simulink model "N3Sim"  (R2023b)
settings: Solver=FixedStepAuto  StartTime=0.0  StopTime=1.04  RelTol=1e-3
values from neighbouring files (symbols this model uses):
  kd = -0.0005    [N3Parameters.m]
  td = 0.01    [N3Parameters.m]
  tl1 = 0.0000199    (= 1.99e-05)    [N3Parameters.m]
  tl2 = 0.0000121    (= 1.21e-05)    [N3Parameters.m]
settings Model: Creator=olavhegg  LastModifiedBy=olavhegg

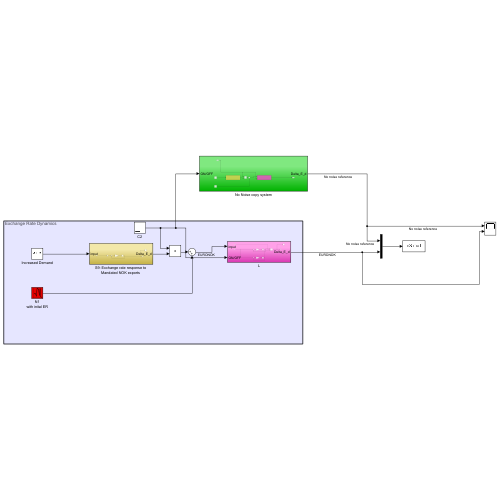
[thumbnail: Simulink's stored preview of the top-level diagram]
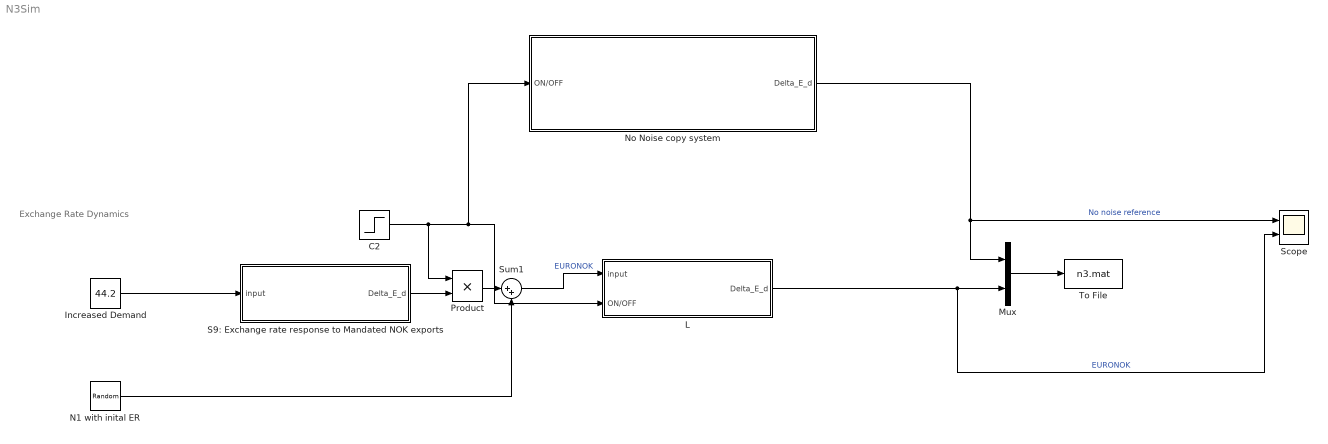
== system N3Sim ==
  note: Exchange Rate Dynamics
  C2 : Step  Time=0.1  SampleTime=0
  Increased Demand : Constant  Value=44.2
  L : Subsystem
  Mux : Mux  Inputs=2
  N1 with inital ER : RandomNumber  Mean=12  Variance=0.00001259  Seed=23341  SampleTime=0.00142857
  No Noise copy system : Subsystem
  Product : Product
  "S9: Exchange rate response to Mandated NOK exports " : Subsystem
  Scope : Scope  NumInputPorts=2
  Sum1 : Sum  Inputs=|++
  To File : ToFile  Filename=n3.mat  MatrixName=n3  SampleTime=0.0001
  wires:
  Product/1 -> Sum1/1
  N1 with inital ER/1 -> Sum1/2
  Sum1/1 -> L/1(input)  "EURONOK"
  No Noise copy system/1(Delta_E_d) -> Mux/1, Scope/1  "No noise reference"
  Mux/1 -> To File/1
  "S9: Exchange rate response to Mandated NOK exports "/1(Delta_E_d) -> Product/2
  C2/1 -> No Noise copy system/1(ON/OFF), L/2(ON/OFF), Product/1
  Increased Demand/1 -> "S9: Exchange rate response to Mandated NOK exports "/1(input)
  L/1(Delta_E_d) -> Scope/2, Mux/2  "EURONOK"

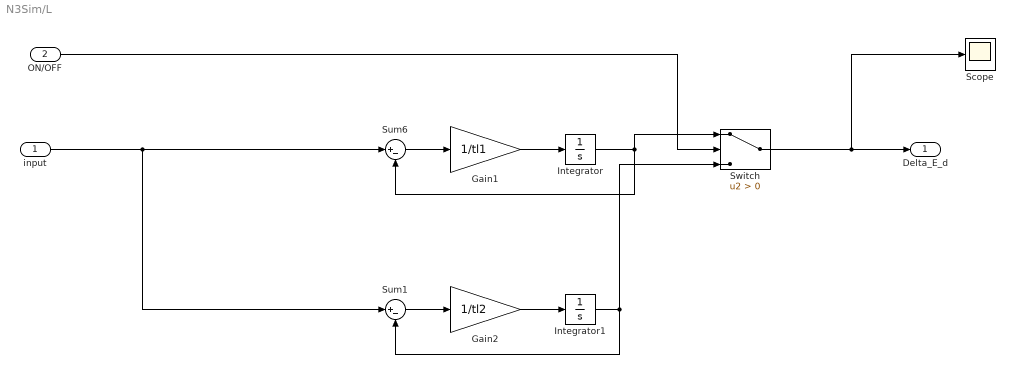
== system N3Sim/L ==
  input : Inport
  ON/OFF : Inport  Port=2
  Gain1 : Gain  Gain=1/tl1
  Gain2 : Gain  Gain=1/tl2
  Integrator : Integrator  InitialCondition=12
  Integrator1 : Integrator  InitialCondition=12
  Scope : Scope
  Sum1 : Sum  Inputs=|+-
  Sum6 : Sum  Inputs=|+-
  Switch : Switch  Criteria=u2 > Threshold  SaturateOnIntegerOverflow=off  InputSameDT=off
  Delta_E_d : Outport
  wires:
  Gain1/1 -> Integrator/1
  Sum6/1 -> Gain1/1
  Integrator/1 -> Switch/1, Sum6/2
  Integrator1/1 -> Switch/3, Sum1/2
  input/1 -> Sum1/1, Sum6/1
  Sum1/1 -> Gain2/1
  Gain2/1 -> Integrator1/1
  Switch/1 -> Scope/1, Delta_E_d/1
  ON/OFF/1 -> Switch/2

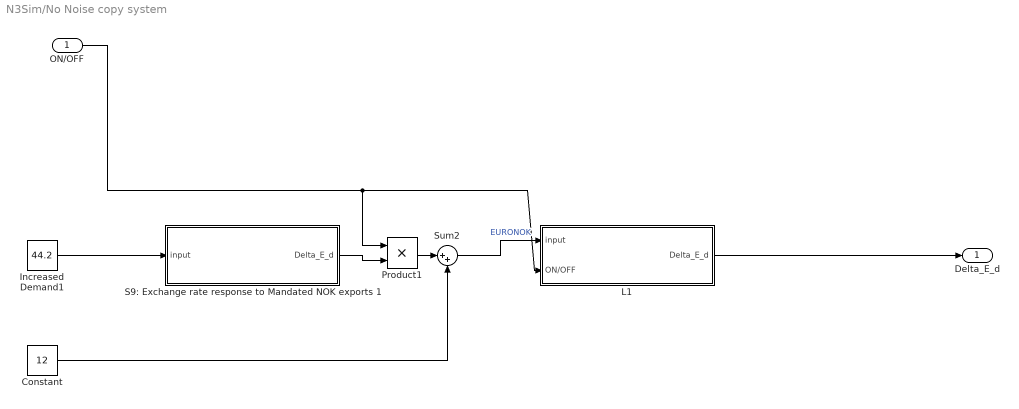
== system N3Sim/No Noise copy system ==
  ON/OFF : Inport
  Constant : Constant  Value=12
  Increased Demand1 : Constant  Value=44.2
  L1 : Subsystem
  Product1 : Product
  S9: Exchange rate response to Mandated NOK exports 1 : Subsystem
  Sum2 : Sum  Inputs=|++
  Delta_E_d : Outport
  wires:
  Increased Demand1/1 -> S9: Exchange rate response to Mandated NOK exports 1/1(input)
  ON/OFF/1 -> L1/2(ON/OFF), Product1/1
  Product1/1 -> Sum2/1
  L1/1(Delta_E_d) -> Delta_E_d/1
  Sum2/1 -> L1/1(input)  "EURONOK"
  Constant/1 -> Sum2/2
  S9: Exchange rate response to Mandated NOK exports 1/1(Delta_E_d) -> Product1/2

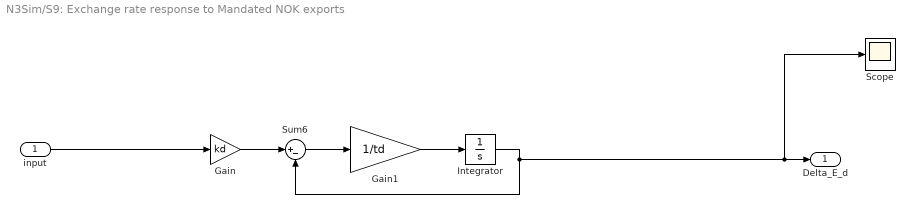
== system N3Sim/S9: Exchange rate response to Mandated NOK exports  ==
  input : Inport
  Gain : Gain  Gain=kd
  Gain1 : Gain  Gain=1/td
  Integrator : Integrator
  Scope : Scope
  Sum6 : Sum  Inputs=|+-
  Delta_E_d : Outport
  wires:
  Gain/1 -> Sum6/1
  Gain1/1 -> Integrator/1
  Sum6/1 -> Gain1/1
  input/1 -> Gain/1
  Integrator/1 -> Scope/1, Delta_E_d/1, Sum6/2

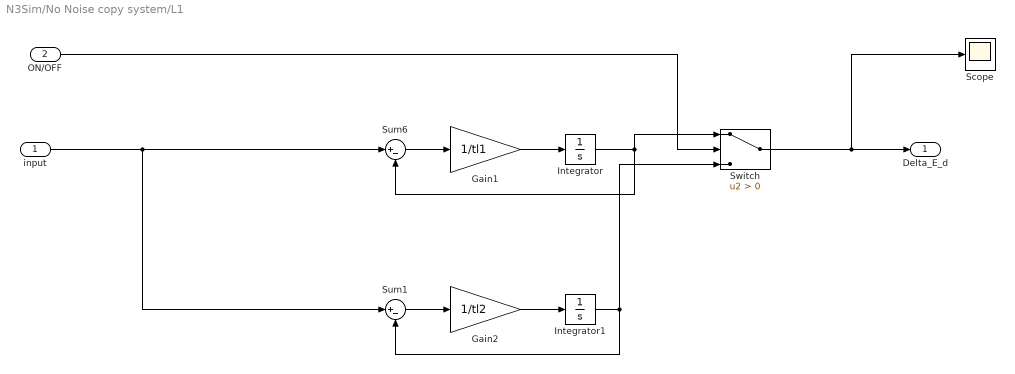
== system N3Sim/No Noise copy system/L1 ==
  input : Inport
  ON/OFF : Inport  Port=2
  Gain1 : Gain  Gain=1/tl1
  Gain2 : Gain  Gain=1/tl2
  Integrator : Integrator  InitialCondition=12
  Integrator1 : Integrator  InitialCondition=12
  Scope : Scope
  Sum1 : Sum  Inputs=|+-
  Sum6 : Sum  Inputs=|+-
  Switch : Switch  Criteria=u2 > Threshold  SaturateOnIntegerOverflow=off  InputSameDT=off
  Delta_E_d : Outport
  wires:
  Gain1/1 -> Integrator/1
  Sum6/1 -> Gain1/1
  Integrator/1 -> Switch/1, Sum6/2
  Integrator1/1 -> Switch/3, Sum1/2
  input/1 -> Sum1/1, Sum6/1
  Sum1/1 -> Gain2/1
  Gain2/1 -> Integrator1/1
  Switch/1 -> Scope/1, Delta_E_d/1
  ON/OFF/1 -> Switch/2

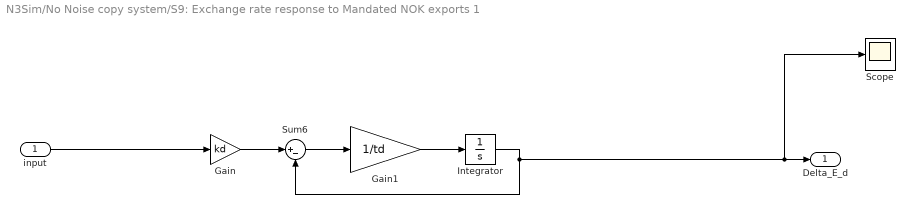
== system N3Sim/No Noise copy system/S9: Exchange rate response to Mandated NOK exports 1 ==
  input : Inport
  Gain : Gain  Gain=kd
  Gain1 : Gain  Gain=1/td
  Integrator : Integrator
  Scope : Scope
  Sum6 : Sum  Inputs=|+-
  Delta_E_d : Outport
  wires:
  Gain/1 -> Sum6/1
  Gain1/1 -> Integrator/1
  Sum6/1 -> Gain1/1
  input/1 -> Gain/1
  Integrator/1 -> Scope/1, Delta_E_d/1, Sum6/2
